simulink model "test"  (R2025b)
settings: Solver=VariableStepAuto  StartTime=0.0  StopTime=10.0  RelTol=1e-3

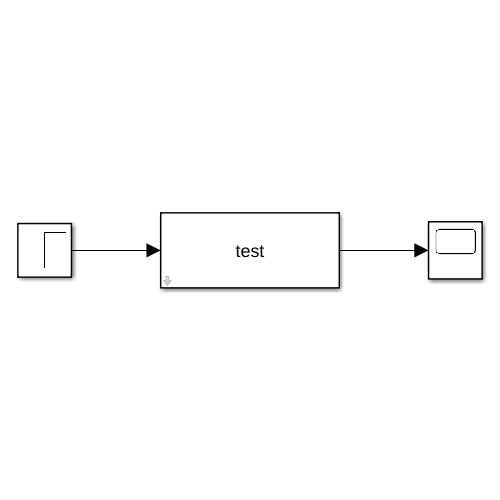
[thumbnail: Simulink's stored preview of the top-level diagram]
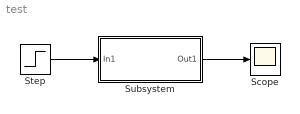
== system test ==
  Scope : Scope
      settings: ActiveDisplayYMinimum=-1.6009281964690314  ActiveDisplayYMaximum=6.3558896633632829
  Step : Step  SampleTime=0
  Subsystem : Subsystem  mask(test){A=1, B=5}
      mask prompts: A "parametrul a"; B "parametrul b"
      mask help: reactie negativa
      mask Help: introdu a si b
      mask Display: disp('test');
  wires:
  Step/1 -> Subsystem/1(In1)
  Subsystem/1(Out1) -> Scope/1

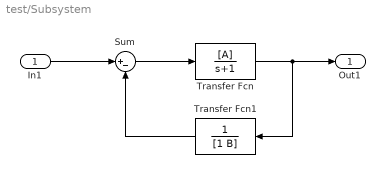
== system test/Subsystem ==
  In1 : Inport
  Sum : Sum  Inputs=|+-
  Transfer Fcn : TransferFcn  Numerator=[A]  Denominator=[1 1]
  Transfer Fcn1 : TransferFcn  Denominator=[1 B]
  Out1 : Outport
  wires:
  In1/1 -> Sum/1
  Transfer Fcn/1 -> Transfer Fcn1/1, Out1/1
  Sum/1 -> Transfer Fcn/1
  Transfer Fcn1/1 -> Sum/2
